simulink model "l9"  (R2015a)
settings: Solver=ode45  StartTime=0.0  StopTime=Tsim  RelTol=1e-3
values from neighbouring files (symbols this model uses):
  C1 = minreal((1/G) * Gcl/(1-Gcl))    [lez9.m]
  C2 = minreal((1/G) * Gcldb/(1-Gcldb))    [lez9.m]
  C3 = minreal((1/Gzero) * Gcl3/(1-Gcl3))    [lez9.m]
  G = 1/((z-0.2)*(z-0.1))    [lez9.m]
  Gzero = K * Gzero    [lez9.m]
  Tc = 0.01    [lez9.m]
settings Model: Creator=lezione  LastModifiedBy=lezione

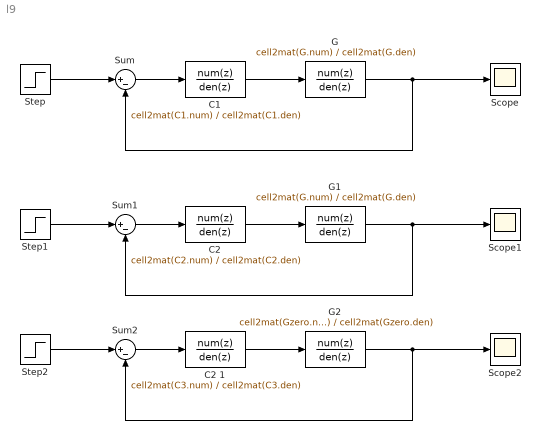
== system l9 ==
  "C1 " : DiscreteTransferFcn  Numerator=cell2mat(C1.num)  Denominator=cell2mat(C1.den)  SampleTime=Tc
  "C2 " : DiscreteTransferFcn  Numerator=cell2mat(C2.num)  Denominator=cell2mat(C2.den)  SampleTime=Tc
  C2 1 : DiscreteTransferFcn  Numerator=cell2mat(C3.num)  Denominator=cell2mat(C3.den)  SampleTime=Tc
  G : DiscreteTransferFcn  Numerator=cell2mat(G.num)  Denominator=cell2mat(G.den)  SampleTime=Tc
  G1 : DiscreteTransferFcn  Numerator=cell2mat(G.num)  Denominator=cell2mat(G.den)  SampleTime=Tc
  G2 : DiscreteTransferFcn  Numerator=cell2mat(Gzero.num)  Denominator=cell2mat(Gzero.den)  SampleTime=Tc
  Scope : Scope
  Scope1 : Scope
  Scope2 : Scope
      settings: SaveName=ScopeData2
  Step : Step  SampleTime=0
  Step1 : Step  SampleTime=0
  Step2 : Step  SampleTime=0
  Sum : Sum  Inputs=|+-
  Sum1 : Sum  Inputs=|+-
  Sum2 : Sum  Inputs=|+-
  wires:
  G/1 -> Sum/2, Scope/1
  "C1 "/1 -> G/1
  Step/1 -> Sum/1
  Sum/1 -> "C1 "/1
  G1/1 -> Sum1/2, Scope1/1
  "C2 "/1 -> G1/1
  Step1/1 -> Sum1/1
  Sum1/1 -> "C2 "/1
  G2/1 -> Sum2/2, Scope2/1
  C2 1/1 -> G2/1
  Step2/1 -> Sum2/1
  Sum2/1 -> C2 1/1
